simulink model "model_for_tsk_3"  (R2015a)
settings: Solver=ode3  StartTime=0.0  StopTime=50  FixedStep=Ts  RelTol=1e-3
settings Model: Creator=chris  LastModifiedBy=chris

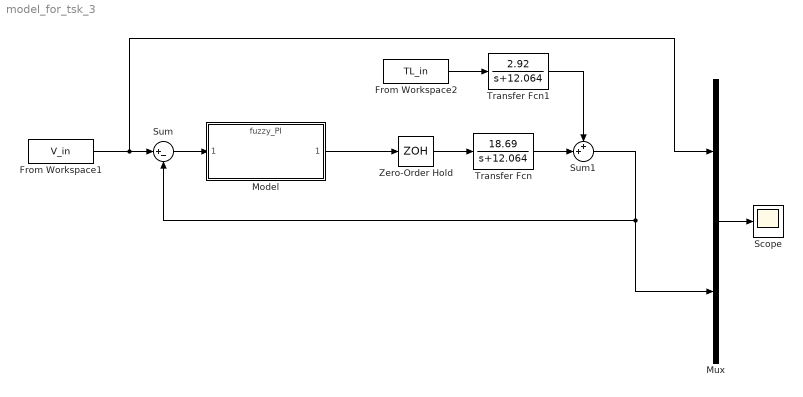
== system model_for_tsk_3 ==
  From Workspace1 : FromWorkspace  VariableName=V_in  SampleTime=0
  From Workspace2 : FromWorkspace  VariableName=TL_in  SampleTime=0
  Model : ModelReference  ModelNameDialog=fuzzy_PI.slx  SimulationMode=Normal  ModelReferenceVersion=1.14  CopyOfModelName=fuzzy_PI.slx  DefaultDataLogging=on
  Mux : Mux  Inputs=2
  Scope : Scope
      settings: TimeRange=30  YMin=-20  YMax=160
  Sum : Sum  Inputs=|+-
  Sum1 : Sum  Inputs=++|
  Transfer Fcn : TransferFcn  Numerator=[18.69]  Denominator=[1 12.064]
  Transfer Fcn1 : TransferFcn  Numerator=[2.92]  Denominator=[1 12.064]
  Zero-Order Hold : ZeroOrderHold  SampleTime=-1
  wires:
  From Workspace1/1 -> Mux/1, Sum/1
  Sum/1 -> Model/1
  Model/1 -> Zero-Order Hold/1
  Zero-Order Hold/1 -> Transfer Fcn/1
  Mux/1 -> Scope/1
  From Workspace2/1 -> Transfer Fcn1/1
  Transfer Fcn1/1 -> Sum1/1
  Transfer Fcn/1 -> Sum1/2
  Sum1/1 -> Mux/2, Sum/2
